simulink model "EJ3_con_ackerman"  (R2020a)
settings: Solver=VariableStepAuto  StartTime=0.0  StopTime=50  RelTol=1e-3
values from neighbouring files (symbols this model uses):
  c_s = 6*m_s    (= 18000)    [parcial2_panchardo_matlab.m]
undefined symbols (not defined in the file or in its folder): K, kr
libraries: fl_lib x13, nesl_utility x9, simulink x3
settings Model: Creator=Adriana  LastModifiedBy=Adriana

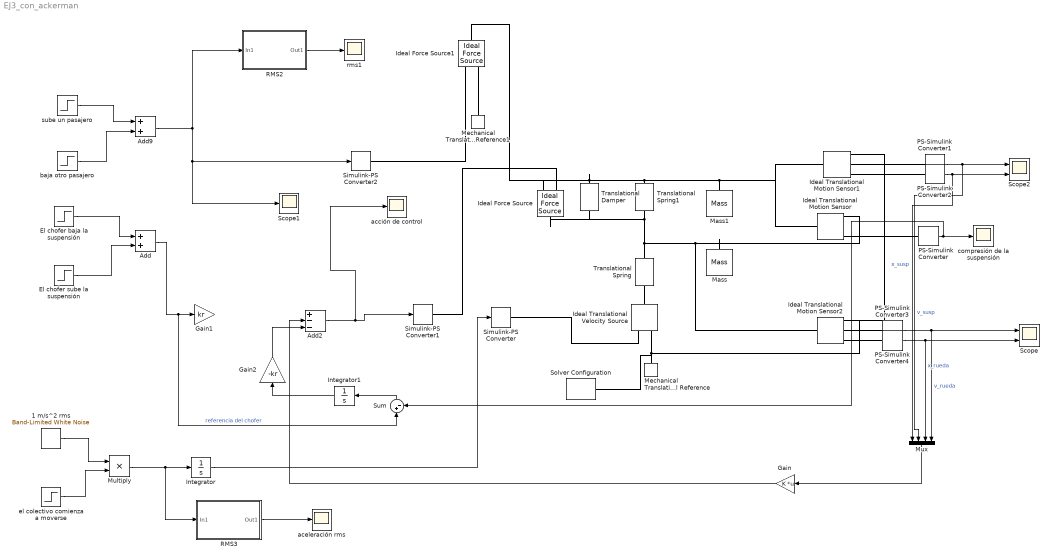
== system EJ3_con_ackerman ==
  1 m/s^2 rms : simulink/Sources/Band-Limited White Noise  Cov=(1^2)/(1/0.1)  Ts=0.1  seed=[98657]
  Add : Sum
  Add2 : Sum  Inputs=+--
  Add9 : Sum
  El chofer baja la suspensión : Step  Time=10  After=-0.10  SampleTime=0
  El chofer sube la suspensión : Step  Time=30  After=.10  SampleTime=0
  Gain : Gain  Gain=K  Multiplication=Matrix(K*u)
  Gain1 : Gain  Gain=kr
  Gain2 : Gain  Gain=-kr
  Ideal Force Source : fl_lib/Mechanical/Mechanical Sources/Ideal Force Source
  Ideal Force Source1 : fl_lib/Mechanical/Mechanical Sources/Ideal Force Source
  Ideal Translational Motion Sensor : fl_lib/Mechanical/Mechanical Sensors/Ideal Translational Motion Sensor  offset=0 m
  Ideal Translational Motion Sensor1 : fl_lib/Mechanical/Mechanical Sensors/Ideal Translational Motion Sensor  offset=0 m
  Ideal Translational Motion Sensor2 : fl_lib/Mechanical/Mechanical Sensors/Ideal Translational Motion Sensor  offset=0 m
  Ideal Translational Velocity Source : fl_lib/Mechanical/Mechanical Sources/Ideal Translational Velocity Source
  Integrator : Integrator
  Integrator1 : Integrator
  Mass : fl_lib/Mechanical/Translational Elements/Mass  mass=m_u kg  v_specify=off  v_priority=High  v=0 m/s  v_nominal_specify=off  v_nominal_unit=m/s  v_nominal_value=1  f_specify=off  f_priority=None  f=0 N  f_nominal_specify=off  f_nominal_unit=N  f_nominal_value=1
  Mass1 : fl_lib/Mechanical/Translational Elements/Mass  mass=m_s kg  v_specify=off  v_priority=High  v=0 m/s  v_nominal_specify=off  v_nominal_unit=m/s  v_nominal_value=1  f_specify=off  f_priority=None  f=0 N  f_nominal_specify=off  f_nominal_unit=N  f_nominal_value=1
  Mechanical Translational Reference : fl_lib/Mechanical/Translational Elements/Mechanical Translational Reference
  Mechanical Translational Reference1 : fl_lib/Mechanical/Translational Elements/Mechanical Translational Reference
  Multiply : Product
  Mux : Mux
  PS-Simulink Converter{,1..4} (5 alike) : nesl_utility/PS-Simulink Converter  PhysicalDomain=network_engine_domain  SubClassName=ps_output  LeftPortType=input  RightPortType=output  PseudoPeriodic=off  Frequencies=[]  Unit=1  AffineConversion=off
  RMS2 : Subsystem
  RMS3 : Subsystem
  Scope : Scope  NumInputPorts=2
  Scope1 : Scope
  Scope2 : Scope  NumInputPorts=2
  Simulink-PS Converter : nesl_utility/Simulink-PS Converter  PhysicalDomain=network_engine_domain  SubClassName=ps_input  LeftPortType=input  RightPortType=output  PseudoPeriodic=off  Frequencies=[]  NoiseDistribution=none  NoiseParameters=[]  Unit=1  AffineConversion=off  FilteringAndDerivatives=provide  SimscapeFilterOrder=1  InputFilterTimeConstant=0.001  UdotUserProvided=0
  Simulink-PS Converter1 : nesl_utility/Simulink-PS Converter  PhysicalDomain=network_engine_domain  SubClassName=ps_input  LeftPortType=input  RightPortType=output  PseudoPeriodic=off  Frequencies=[]  NoiseDistribution=none  NoiseParameters=[]  Unit=1  AffineConversion=off  FilteringAndDerivatives=provide  SimscapeFilterOrder=1  InputFilterTimeConstant=0.001  UdotUserProvided=0
  Simulink-PS Converter2 : nesl_utility/Simulink-PS Converter  PhysicalDomain=network_engine_domain  SubClassName=ps_input  LeftPortType=input  RightPortType=output  PseudoPeriodic=off  Frequencies=[]  NoiseDistribution=none  NoiseParameters=[]  Unit=1  AffineConversion=off  FilteringAndDerivatives=provide  SimscapeFilterOrder=1  InputFilterTimeConstant=0.001  UdotUserProvided=0
  Solver Configuration : nesl_utility/Solver Configuration  PhysicalDomain=network_engine_domain  SubClassName=solver  LeftPortType=input  RightPortType=generic  Tones=[]  Harmonics=[]  SimulateNoise=off  Profile=off  UseLocalSampling=off  EnableSwitchedLinearOptims=on  FrequencyDomain=off  UseCCode=off  RelTol=0.001  AbsTol=1e-06  MinStep=1e-09  ToWorkspace=off  RevertToSquareIcSolve=off  NumHomotopyIterations=100  PhasorMode=off  PhasorModeNumHarmonics=1  DoDC=off  ResidualTolerance=1e-09  UseLocalSolver=off  LocalSolverChoice=NE_BACKWARD_EULER_ADVANCER  LocalSolverSampleTime=0.001  DoFixedCost=off  MaxNonlinIter=3  MaxModeIter=2  LinearAlgebra=Sparse  EquationFormulation=NE_TIME_EF  DelaysMemoryBudget=1024  AutomaticFiltering=on  FilteringTimeConstant=0.001  PartitionStorageMethod=AS_NEEDED  PartitionMemoryBudget=1024  PartitionMethod=FAST
  Sum : Sum  Inputs=|+-
  Translational Damper : fl_lib/Mechanical/Translational Elements/Translational Damper  D=c_s N/(m/s)  v_specify=off  v_priority=None  v=0 m/s  v_nominal_specify=off  v_nominal_unit=m/s  v_nominal_value=1  f_specify=off  f_priority=None  f=0 N  f_nominal_specify=off  f_nominal_unit=N  f_nominal_value=1
  Translational Spring : fl_lib/Mechanical/Translational Elements/Translational Spring  spr_rate=k_t N/m  v_specify=off  v_priority=None  v=0 m/s  v_nominal_specify=off  v_nominal_unit=m/s  v_nominal_value=1  f_specify=off  f_priority=None  f=0 N  f_nominal_specify=off  f_nominal_unit=N  f_nominal_value=1  x_specify=off  x_priority=High  x=0 m  x_nominal_specify=off  x_nominal_unit=m  x_nominal_value=1
  Translational Spring1 : fl_lib/Mechanical/Translational Elements/Translational Spring  spr_rate=k_s N/m  v_specify=off  v_priority=None  v=0 m/s  v_nominal_specify=off  v_nominal_unit=m/s  v_nominal_value=1  f_specify=off  f_priority=None  f=0 N  f_nominal_specify=off  f_nominal_unit=N  f_nominal_value=1  x_specify=off  x_priority=High  x=0 m  x_nominal_specify=off  x_nominal_unit=m  x_nominal_value=1
  acción de control : Scope
  aceleración rms : Scope
  baja otro pasajero : Step  Time=25  After=-700  SampleTime=0
  compresión de la suspensión : Scope
  el colectivo comienza a moverse : Step  Time=50  SampleTime=0
  rms1 : Scope
  sube un pasajero : Step  Time=20  After=700  SampleTime=0
  wires:
  PS-Simulink Converter/1 -> Sum/2, compresión de la suspensión/1
  Integrator/1 -> Simulink-PS Converter/1
  1 m/s^2 rms/1 -> Multiply/1
  RMS3/1(Out1) -> aceleración rms/1
  Multiply/1 -> RMS3/1(In1), Integrator/1
  el colectivo comienza a moverse/1 -> Multiply/2
  Add9/1 -> Scope1/1, Simulink-PS Converter2/1, RMS2/1(In1)
  RMS2/1(Out1) -> rms1/1
  baja otro pasajero/1 -> Add9/2
  sube un pasajero/1 -> Add9/1
  Add/1 -> Gain1/1, Sum/1  "referencia del chofer"
  El chofer baja la suspensión/1 -> Add/1
  El chofer sube la suspensión/1 -> Add/2
  Add2/1 -> acción de control/1, Simulink-PS Converter1/1
  Gain/1 -> Add2/2
  PS-Simulink Converter3/1 -> Scope/1, Mux/4  "v_rueda"
  PS-Simulink Converter4/1 -> Scope/2, Mux/3  "x_rueda"
  PS-Simulink Converter1/1 -> Mux/2, Scope2/1  "v_susp"
  PS-Simulink Converter2/1 -> Mux/1, Scope2/2  "x_susp"
  Mux/1 -> Gain/1
  Gain2/1 -> Add2/3
  Sum/1 -> Integrator1/1
  Integrator1/1 -> Gain2/1
  connections:
  Solver Configuration/RConn1 -- Ideal Translational Motion Sensor1/RConn1 -- Ideal Translational Motion Sensor2/RConn1 -- Mechanical Translational Reference/LConn1 -- Ideal Translational Velocity Source/RConn2
  PS-Simulink Converter/LConn1 -- Ideal Translational Motion Sensor/RConn3
  Mechanical Translational Reference1/LConn1 -- Ideal Force Source1/RConn2
  Ideal Translational Velocity Source/LConn1 -- Translational Spring/RConn1
  Translational Spring/LConn1 -- Ideal Translational Motion Sensor2/LConn1 -- Ideal Translational Motion Sensor/RConn1 -- Mass/LConn1 -- Ideal Force Source/LConn1 -- Translational Damper/RConn1 -- Translational Spring1/RConn1
  Mass1/LConn1 -- Ideal Translational Motion Sensor/LConn1 -- Ideal Translational Motion Sensor1/LConn1 -- Ideal Force Source1/LConn1 -- Ideal Force Source/RConn2 -- Translational Damper/LConn1 -- Translational Spring1/LConn1
  Simulink-PS Converter/RConn1 -- Ideal Translational Velocity Source/RConn1
  Simulink-PS Converter2/RConn1 -- Ideal Force Source1/RConn1
  Simulink-PS Converter1/RConn1 -- Ideal Force Source/RConn1
  PS-Simulink Converter1/LConn1 -- Ideal Translational Motion Sensor1/RConn2
  PS-Simulink Converter2/LConn1 -- Ideal Translational Motion Sensor1/RConn3
  PS-Simulink Converter3/LConn1 -- Ideal Translational Motion Sensor2/RConn2
  Ideal Translational Motion Sensor2/RConn3 -- PS-Simulink Converter4/LConn1

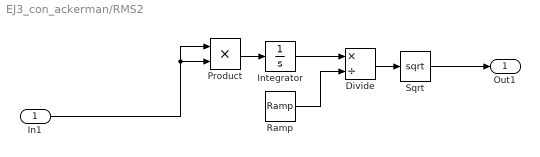
== system EJ3_con_ackerman/RMS2 ==
  In1 : Inport
  Divide : Product  Inputs=*/
  Integrator : Integrator
  Product : Product
  Ramp : simulink/Sources/Ramp  slope=1  start=0  InitialOutput=0
  Sqrt : Sqrt  SaturateOnIntegerOverflow=on
  Out1 : Outport  VectorParamsAs1DForOutWhenUnconnected=off
  wires:
  Ramp/1 -> Divide/2
  Product/1 -> Integrator/1
  Integrator/1 -> Divide/1
  Sqrt/1 -> Out1/1
  Divide/1 -> Sqrt/1
  In1/1 -> Product/1, Product/2

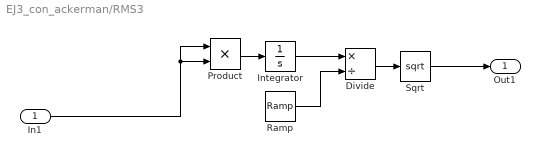
== system EJ3_con_ackerman/RMS3 ==
  In1 : Inport
  Divide : Product  Inputs=*/
  Integrator : Integrator
  Product : Product
  Ramp : simulink/Sources/Ramp  slope=1  start=0  InitialOutput=0
  Sqrt : Sqrt  SaturateOnIntegerOverflow=on
  Out1 : Outport  VectorParamsAs1DForOutWhenUnconnected=off
  wires:
  Ramp/1 -> Divide/2
  Product/1 -> Integrator/1
  Integrator/1 -> Divide/1
  Sqrt/1 -> Out1/1
  Divide/1 -> Sqrt/1
  In1/1 -> Product/1, Product/2
